simulink model "MathWithData"  (R2015b)
settings: Solver=VariableStepAuto  StartTime=0.0  StopTime=inf  RelTol=1e-3
settings Model: Creator=Druzhinin_Vasily  LastModifiedBy=Druzhinin_Vasily

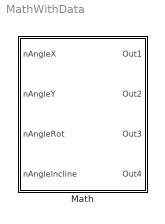
== system MathWithData ==
  Math : Subsystem

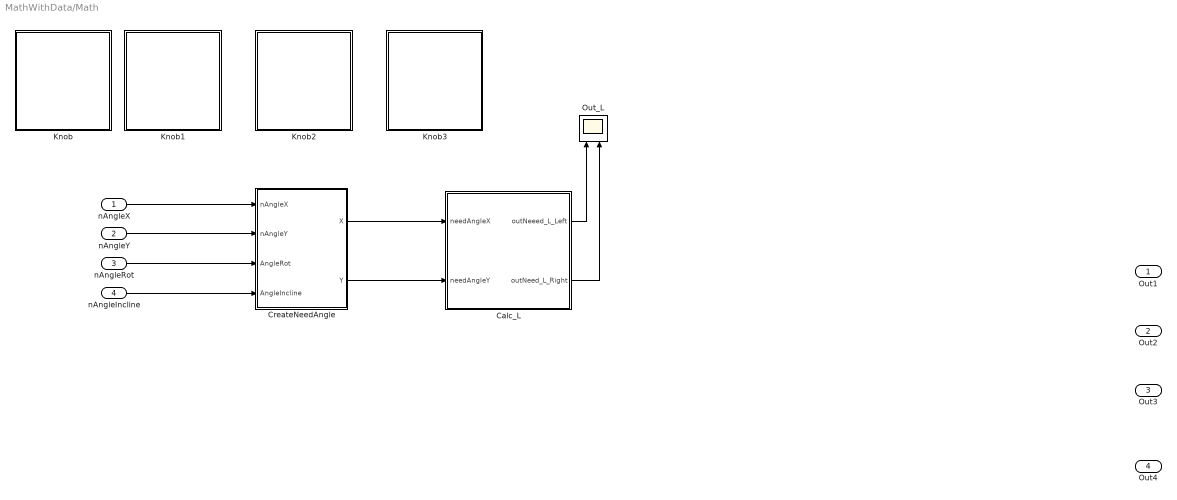
== system MathWithData/Math ==
  nAngleX : Inport
  nAngleY : Inport  Port=2
  nAngleRot : Inport  Port=3
  nAngleIncline : Inport  Port=4
  Calc_L : MATLAB Function  TreatAsAtomicUnit=on
  CreateNeedAngle : Subsystem
  Knob : Subsystem  DialogController=hmiCreateDDGDialog  IsWebBlock=on  mask(MWDashboardBlock){webBlockId=64e31e70-0dc6-4a47-9a86-7618526540fd, webBlockType=continuousknob, ShowInLibBrowser=on, ShowInitialText=on, HMISrcModelName=MathWithData}
      mask prompts: webBlockId "WebBlock Id"; webBlockType "WebBlock Type"; HMISrcModelName "Source Model"
      mask Help: helpview([docroot '/mapfiles/simulink.map'], 'hmi_knob')
      mask Display:
      | if strcmp(get_param(bdroot(gcb),'BlockDiagramType'), 'library')
      |     image([(matlabroot) '/toolbox/simulink/hmi/icons/ContinuousKnob.png']);
      | end
  Knob1 : Subsystem  DialogController=hmiCreateDDGDialog  IsWebBlock=on  mask(MWDashboardBlock){webBlockId=c3abfad3-0788-43a3-9b1c-e570a5e0faec, webBlockType=continuousknob, ShowInLibBrowser=on, ShowInitialText=on, HMISrcModelName=MathWithData}
      mask prompts: webBlockId "WebBlock Id"; webBlockType "WebBlock Type"; HMISrcModelName "Source Model"
      mask Help: helpview([docroot '/mapfiles/simulink.map'], 'hmi_knob')
      mask Display:
      | if strcmp(get_param(bdroot(gcb),'BlockDiagramType'), 'library')
      |     image([(matlabroot) '/toolbox/simulink/hmi/icons/ContinuousKnob.png']);
      | end
  Knob2 : Subsystem  DialogController=hmiCreateDDGDialog  IsWebBlock=on  mask(MWDashboardBlock){webBlockId=5ab4cb30-d487-4d68-876b-1200134c20e5, webBlockType=continuousknob, ShowInLibBrowser=on, ShowInitialText=on, HMISrcModelName=MathWithData}
      mask prompts: webBlockId "WebBlock Id"; webBlockType "WebBlock Type"; HMISrcModelName "Source Model"
      mask Help: helpview([docroot '/mapfiles/simulink.map'], 'hmi_knob')
      mask Display:
      | if strcmp(get_param(bdroot(gcb),'BlockDiagramType'), 'library')
      |     image([(matlabroot) '/toolbox/simulink/hmi/icons/ContinuousKnob.png']);
      | end
  Knob3 : Subsystem  DialogController=hmiCreateDDGDialog  IsWebBlock=on  mask(MWDashboardBlock){webBlockId=efa038c8-923f-40da-8967-e9d77197a2d3, webBlockType=continuousknob, ShowInLibBrowser=on, ShowInitialText=on, HMISrcModelName=MathWithData}
      mask prompts: webBlockId "WebBlock Id"; webBlockType "WebBlock Type"; HMISrcModelName "Source Model"
      mask Help: helpview([docroot '/mapfiles/simulink.map'], 'hmi_knob')
      mask Display:
      | if strcmp(get_param(bdroot(gcb),'BlockDiagramType'), 'library')
      |     image([(matlabroot) '/toolbox/simulink/hmi/icons/ContinuousKnob.png']);
      | end
  Out_L : Scope  NumInputPorts=2
  Out1 : Outport
  Out2 : Outport  Port=2
  Out3 : Outport  Port=3
  Out4 : Outport  Port=4
  wires:
  Calc_L/1(outNeeed_L_Left) -> Out_L/1
  Calc_L/2(outNeed_L_Right) -> Out_L/2
  CreateNeedAngle/1(X) -> Calc_L/1(needAngleX)
  CreateNeedAngle/2(Y) -> Calc_L/2(needAngleY)
  nAngleX/1 -> CreateNeedAngle/1(nAngleX)
  nAngleY/1 -> CreateNeedAngle/2(nAngleY)
  nAngleRot/1 -> CreateNeedAngle/3(AngleRot)
  nAngleIncline/1 -> CreateNeedAngle/4(AngleIncline)

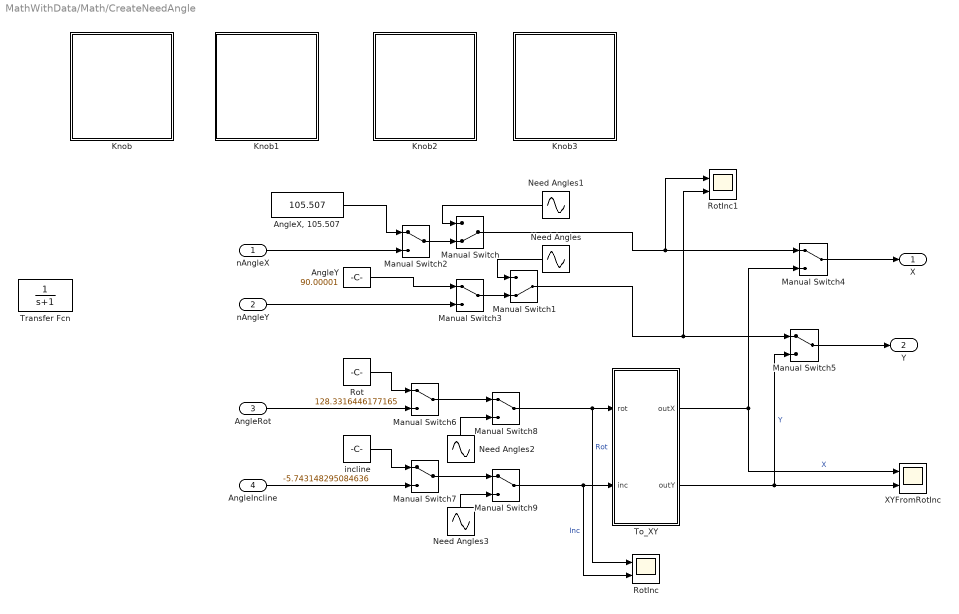
== system MathWithData/Math/CreateNeedAngle ==
  nAngleX : Inport
  nAngleY : Inport  Port=2
  AngleRot : Inport  Port=3
  AngleIncline : Inport  Port=4
  "AngleX, 105.507" : Constant  Value=105.507
  AngleY : Constant  Value=90.00001
  Knob : Subsystem  DialogController=hmiCreateDDGDialog  IsWebBlock=on  mask(MWDashboardBlock){webBlockId=e22f60da-0c24-433e-8a33-0987d0b779e5, webBlockType=continuousknob, ShowInLibBrowser=on, ShowInitialText=on, HMISrcModelName=MathWithData}
      mask prompts: webBlockId "WebBlock Id"; webBlockType "WebBlock Type"; HMISrcModelName "Source Model"
      mask Help: helpview([docroot '/mapfiles/simulink.map'], 'hmi_knob')
      mask Display:
      | if strcmp(get_param(bdroot(gcb),'BlockDiagramType'), 'library')
      |     image([(matlabroot) '/toolbox/simulink/hmi/icons/ContinuousKnob.png']);
      | end
  Knob1 : Subsystem  DialogController=hmiCreateDDGDialog  IsWebBlock=on  mask(MWDashboardBlock){webBlockId=c64beda5-346f-4528-877c-0d7d0d130db5, webBlockType=continuousknob, ShowInLibBrowser=on, ShowInitialText=on, HMISrcModelName=MathWithData}
      mask prompts: webBlockId "WebBlock Id"; webBlockType "WebBlock Type"; HMISrcModelName "Source Model"
      mask Help: helpview([docroot '/mapfiles/simulink.map'], 'hmi_knob')
      mask Display:
      | if strcmp(get_param(bdroot(gcb),'BlockDiagramType'), 'library')
      |     image([(matlabroot) '/toolbox/simulink/hmi/icons/ContinuousKnob.png']);
      | end
  Knob2 : Subsystem  DialogController=hmiCreateDDGDialog  IsWebBlock=on  mask(MWDashboardBlock){webBlockId=ddfa458b-8b5c-4f60-9831-3ad83f2b0118, webBlockType=continuousknob, ShowInLibBrowser=on, ShowInitialText=on, HMISrcModelName=MathWithData}
      mask prompts: webBlockId "WebBlock Id"; webBlockType "WebBlock Type"; HMISrcModelName "Source Model"
      mask Help: helpview([docroot '/mapfiles/simulink.map'], 'hmi_knob')
      mask Display:
      | if strcmp(get_param(bdroot(gcb),'BlockDiagramType'), 'library')
      |     image([(matlabroot) '/toolbox/simulink/hmi/icons/ContinuousKnob.png']);
      | end
  Knob3 : Subsystem  DialogController=hmiCreateDDGDialog  IsWebBlock=on  mask(MWDashboardBlock){webBlockId=a02248f1-13d5-45be-9288-4bb0111df98c, webBlockType=continuousknob, ShowInLibBrowser=on, ShowInitialText=on, HMISrcModelName=MathWithData}
      mask prompts: webBlockId "WebBlock Id"; webBlockType "WebBlock Type"; HMISrcModelName "Source Model"
      mask Help: helpview([docroot '/mapfiles/simulink.map'], 'hmi_knob')
      mask Display:
      | if strcmp(get_param(bdroot(gcb),'BlockDiagramType'), 'library')
      |     image([(matlabroot) '/toolbox/simulink/hmi/icons/ContinuousKnob.png']);
      | end
  Manual Switch : ManualSwitch  CurrentSetting=0
  Manual Switch1 : ManualSwitch  CurrentSetting=0
  Manual Switch{2..9} (8 alike) : ManualSwitch
  Need Angles : Sin  Amplitude=20  Bias=90  SampleTime=0
  Need Angles1 : Sin  Amplitude=10  Bias=90  SampleTime=0
  Need Angles2 : Sin  Amplitude=360  Bias=180  SampleTime=0
  Need Angles3 : Sin  Amplitude=10  Bias=90  SampleTime=0
  Rot : Constant  Value=128.3316446177165
  RotInc : Scope  NumInputPorts=2
  RotInc1 : Scope  NumInputPorts=2
  To_XY : MATLAB Function  TreatAsAtomicUnit=on
  Transfer Fcn : TransferFcn  Denominator=[1 1]
  XYFromRotInc : Scope  NumInputPorts=2
  incline : Constant  Value=-5.743148295084636
  X : Outport
  Y : Outport  Port=2
  wires:
  Need Angles/1 -> Manual Switch1/1
  Need Angles1/1 -> Manual Switch/1
  Manual Switch2/1 -> Manual Switch/2
  Manual Switch3/1 -> Manual Switch1/2
  "AngleX, 105.507"/1 -> Manual Switch2/1
  AngleY/1 -> Manual Switch3/1
  nAngleX/1 -> Manual Switch2/2
  nAngleY/1 -> Manual Switch3/2
  Manual Switch4/1 -> X/1
  Manual Switch/1 -> RotInc1/1, Manual Switch4/1
  Manual Switch5/1 -> Y/1
  Manual Switch1/1 -> RotInc1/2, Manual Switch5/1
  Rot/1 -> Manual Switch6/1
  AngleRot/1 -> Manual Switch6/2
  incline/1 -> Manual Switch7/1
  AngleIncline/1 -> Manual Switch7/2
  Manual Switch7/1 -> Manual Switch9/1
  Manual Switch6/1 -> Manual Switch8/1
  Need Angles2/1 -> Manual Switch8/2
  Need Angles3/1 -> Manual Switch9/2
  To_XY/1(outX) -> XYFromRotInc/1, Manual Switch4/2  "X"
  Manual Switch8/1 -> To_XY/1(rot), RotInc/1  "Rot"
  Manual Switch9/1 -> To_XY/2(inc), RotInc/2  "Inc"
  To_XY/2(outY) -> Manual Switch5/2, XYFromRotInc/2  "Y"

== system MathWithData/Math/Knob ==

== system MathWithData/Math/Knob1 ==

== system MathWithData/Math/Knob2 ==

== system MathWithData/Math/Knob3 ==

== system MathWithData/Math/CreateNeedAngle/Knob ==

== system MathWithData/Math/CreateNeedAngle/Knob1 ==

== system MathWithData/Math/CreateNeedAngle/Knob2 ==

== system MathWithData/Math/CreateNeedAngle/Knob3 ==

== matlab function MathWithData/Math/CreateNeedAngle/To_XY ==
  data: rot input; outX output; inc input; outY output
function [outX,outY] = fcn(rot,inc)
rotR = GradToRad(rot);
incR = GradToRad(inc);


if (rot == 0)
    X = inc;
    Y = 90;
elseif (rot>0)&&(rot<90)%1
    X = inc*cos(rotR);
    Y = inc*sin(rotR);
elseif (rot==90)
    X=90;
    Y=inc;
elseif (rot>90)&&(rot<180) %2
    rotR = rotR - GradToRad(90);
    X = inc*sin(rotR);
    Y = inc*cos(rotR);
elseif (rot==180)
    X = inc;
    Y = 90;
elseif (rot>180) &&(rot<270)%3
    rotR = rotR - GradToRad(180);
    X = inc*cos(rotR);
    Y = inc*sin(rotR);
elseif (rot==270)
    X=90;
    Y=inc;
else %4
    rotR = rotR - GradToRad(270);
    X = inc*sin(rotR);
    Y = inc*cos(rotR);
end
    outX = 90 + X;
    outY = 90 + Y;

== matlab function MathWithData/Math/Calc_L ==
  data: needAngleX input; outNeeed_L_Left output; needAngleY input; outNeed_L_Right output
function [outNeeed_L_Left,outNeed_L_Right] = fcn(needAngleX,needAngleY)
%#codegen

%Data
aX = 171.50;
bX = 448.84;

a = 139.5;
k = 76.5;
aY = a - k;
bY = 432.5;

startL = 539.85;


%CalcL
L_fromOZD_Left_X  = Calc_L_UndoAlfa(aX,bX,needAngleX);
L_fromOZD_Right_X = Calc_L_UndoAlfa(aX,bX,needAngleX);

if (needAngleY<90)
    
    L_fromOZD_Left_Y  = startL - Calc_L_UndoAlfa(aY,bY,needAngleY);
    L_fromOZD_Right_Y = -1 *(startL - Calc_L_UndoAlfa(aY,bY,needAngleY));
    
elseif (needAngleY>90)
        
    L_fromOZD_Left_Y  = -1 * (startL - Calc_L_UndoAlfa(aY,bY,needAngleY));
    L_fromOZD_Right_Y = startL - Calc_L_UndoAlfa(aY,bY,needAngleY);
    
else
    L_fromOZD_Left_Y  = 0;
    L_fromOZD_Right_Y = 0;
end;
    

outNeeed_L_Left = L_fromOZD_Left_X + L_fromOZD_Left_Y;
outNeed_L_Right = L_fromOZD_Right_X + L_fromOZD_Right_Y;
